simulink model "PF70mmDuctFanN"  (R2018b)
settings: Solver=FixedStepAuto  StartTime=0.0  StopTime=10.0  RelTol=1e-3
libraries: simulink x1, vrlib x1
settings Model: Creator=sweat  LastModifiedBy=39926

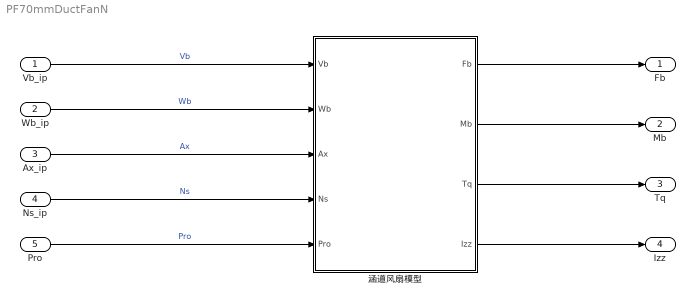
== system PF70mmDuctFanN ==
  Vb_ip : Inport  PortDimensions=3
  Wb_ip : Inport  Port=2  PortDimensions=3
  Ax_ip : Inport  Port=3  PortDimensions=3
  Ns_ip : Inport  Port=4  PortDimensions=1
  Pro : Inport  Port=5  PortDimensions=1
  "涵道风扇模型 " : Subsystem  mask{Fratio=1.016, Mratio=1.24, Izz=0.00000309}
      mask prompts: Fratio "涵道风扇气动力修正系数"; Mratio "涵道风扇气动力矩修正系数"; Izz "涵道风扇转动惯量"
  Fb : Outport
  Mb : Outport  Port=2
  Tq : Outport  Port=3
  Izz : Outport  Port=4
  wires:
  Vb_ip/1 -> "涵道风扇模型 "/1(Vb)  "Vb"
  Wb_ip/1 -> "涵道风扇模型 "/2(Wb)  "Wb"
  Ax_ip/1 -> "涵道风扇模型 "/3(Ax)  "Ax"
  Ns_ip/1 -> "涵道风扇模型 "/4(Ns)  "Ns"
  Pro/1 -> "涵道风扇模型 "/5(Pro)  "Pro"
  "涵道风扇模型 "/1(Fb) -> Fb/1
  "涵道风扇模型 "/2(Mb) -> Mb/1
  "涵道风扇模型 "/3(Tq) -> Tq/1
  "涵道风扇模型 "/4(Izz) -> Izz/1

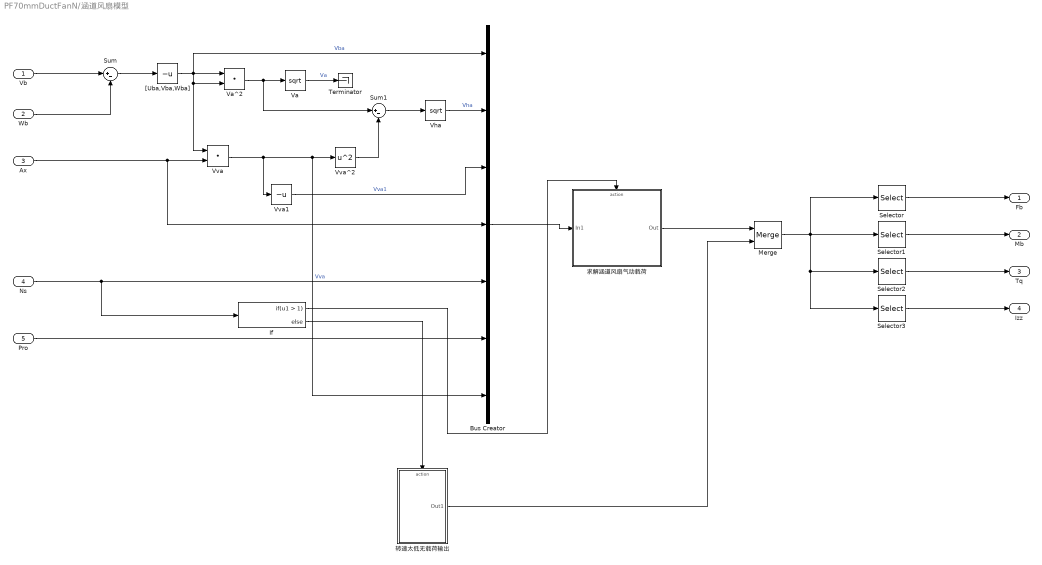
== system PF70mmDuctFanN/涵道风扇模型  ==
  Vb : Inport
  Wb : Inport  Port=2
  Ax : Inport  Port=3
  Ns : Inport  Port=4
  Pro : Inport  Port=5
  Bus Creator : BusCreator  Inputs=7
  If : If  IfExpression=u1 > 1
  Merge : Merge
  Selector : Selector  InputPortWidth=8  IndexOptions=Index vector (dialog)  Indices=[1:3]  OutputSizes=1
  Selector1 : Selector  InputPortWidth=8  IndexOptions=Index vector (dialog)  Indices=[4:6]  OutputSizes=1
  Selector2 : Selector  InputPortWidth=8  IndexOptions=Index vector (dialog)  Indices=[7]  OutputSizes=1
  Selector3 : Selector  InputPortWidth=8  IndexOptions=Index vector (dialog)  Indices=8  OutputSizes=1
  Sum : Sum  Inputs=|+-
  Sum1 : Sum  Inputs=|+-
  Terminator : Terminator
  Va : Sqrt  SaturateOnIntegerOverflow=on
  Va^2 : DotProduct  InputSameDT=on  OutDataTypeStr=Inherit: Inherit via internal rule
  Vha : Sqrt  SaturateOnIntegerOverflow=on
  Vva : DotProduct  InputSameDT=on  OutDataTypeStr=Inherit: Inherit via internal rule
  Vva1 : UnaryMinus
  Vva^2 : Math  Operator=square  SaturateOnIntegerOverflow=on
  "[Uba,Vba,Wba]" : UnaryMinus
  求解涵道风扇气动载荷 : Subsystem  TreatAsAtomicUnit=on
  转速太低无载荷输出 : Subsystem  TreatAsAtomicUnit=on
  Fb : Outport
  Mb : Outport  Port=2
  Tq : Outport  Port=3
  Izz : Outport  Port=4
  wires:
  Vb/1 -> Sum/1
  Wb/1 -> Sum/2
  Sum/1 -> "[Uba,Vba,Wba]"/1
  "[Uba,Vba,Wba]"/1 -> Bus Creator/1, Vva/1, Va^2/2, Va^2/1  "Vba"
  Ax/1 -> Bus Creator/4, Vva/2
  Va^2/1 -> Sum1/1, Va/1
  Vva/1 -> Bus Creator/7, Vva^2/1, Vva1/1  "Vva"
  Vva^2/1 -> Sum1/2
  Sum1/1 -> Vha/1
  Vha/1 -> Bus Creator/2  "Vha"
  Vva1/1 -> Bus Creator/3  "Vva1"
  Ns/1 -> Bus Creator/5, If/1
  If/1 -> 求解涵道风扇气动载荷/Action
  If/2 -> 转速太低无载荷输出/Action
  Pro/1 -> Bus Creator/6
  Bus Creator/1 -> 求解涵道风扇气动载荷/1(In1)
  Va/1 -> Terminator/1  "Va"
  Merge/1 -> Selector3/1, Selector2/1, Selector1/1, Selector/1
  求解涵道风扇气动载荷/1(Out) -> Merge/1
  转速太低无载荷输出/1(Out1) -> Merge/2
  Selector/1 -> Fb/1
  Selector1/1 -> Mb/1
  Selector2/1 -> Tq/1
  Selector3/1 -> Izz/1

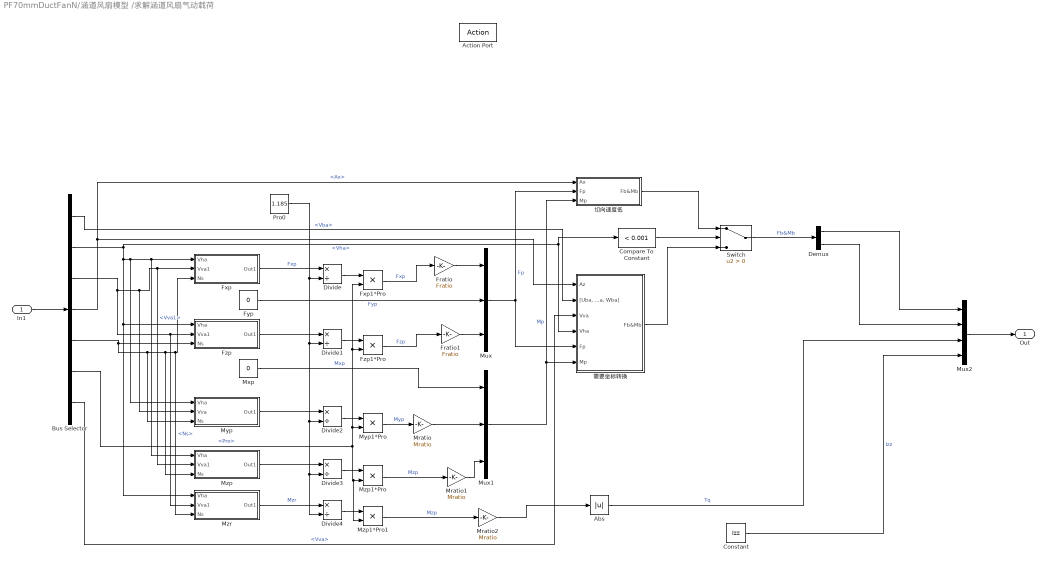
== system PF70mmDuctFanN/涵道风扇模型 /求解涵道风扇气动载荷 ==
  In1 : Inport
  Action Port : ActionPort  ActionType=then
  Abs : Abs
  Bus Selector : BusSelector  OutputSignals=Vba,Vha,Vva1,Ax,Ns,Pro,Vva
  Compare To Constant : simulink/Logic and Bit Operations/Compare To Constant  relop=<  const=0.001  OutDataTypeStr=boolean
  Constant : Constant  Value=Izz
  Demux : Demux  Outputs=2
  Divide{,1..4} (5 alike) : Product  Inputs=*/
  Fratio : Gain  Gain=Fratio
  Fratio1 : Gain  Gain=Fratio
  Fxp : Subsystem
  Fxp1*Pro : Product
  Fyp : Constant  Value=0
  Fzp : Subsystem
  Fzp1*Pro : Product
  Mratio : Gain  Gain=Mratio
  Mratio1 : Gain  Gain=Mratio
  Mratio2 : Gain  Gain=Mratio
  Mux : Mux  Inputs=3
  Mux1 : Mux  Inputs=3
  Mux2 : Mux
  Mxp : Constant  Value=0
  Myp : Subsystem
  Myp1*Pro : Product
  Mzp : Subsystem
  Mzp1*Pro : Product
  Mzp1*Pro1 : Product
  Mzr : Subsystem
  Pro0 : Constant  Value=1.185
  Switch : Switch  Criteria=u2 > Threshold
  切向速度低 : Subsystem
  需要坐标转换 : Subsystem
  Out : Outport
  wires:
  In1/1 -> Bus Selector/1
  Bus Selector/2 -> Mzr/1(Vha), Fzp/1(Vha), Myp/1(Vha), Mzp/1(Vha), Fxp/1(Vha), 需要坐标转换/4(Vha), Compare To Constant/1  "<Vha>"
  Bus Selector/3 -> Myp/2(Vva), Mzp/2(Vva1), Fxp/2(Vva1), Mzr/2(Vva1), Fzp/2(Vva1)  "<Vva1>"
  Bus Selector/5 -> Fzp/3(Ns), Myp/3(Ns), Mzp/3(Ns), Mzr/3(Ns), Fxp/3(Ns)  "<Ns>"
  Fyp/1 -> Mux/2  "Fyp"
  Fxp/1(Out1) -> Divide/1  "Fxp"
  Fzp/1(Out1) -> Divide1/1
  Myp/1(Out1) -> Divide2/1
  Mzp/1(Out1) -> Divide3/1
  Pro0/1 -> Divide4/2, Divide3/2, Divide2/2, Divide1/2, Divide/2
  Divide/1 -> Fxp1*Pro/1
  Fxp1*Pro/1 -> Fratio/1  "Fxp"
  Divide1/1 -> Fzp1*Pro/1
  Fzp1*Pro/1 -> Fratio1/1  "Fzp"
  Bus Selector/6 -> Mzp1*Pro1/2, Mzp1*Pro/2, Myp1*Pro/2, Fzp1*Pro/2, Fxp1*Pro/2  "<Pro>"
  Divide2/1 -> Myp1*Pro/1
  Myp1*Pro/1 -> Mratio/1  "Myp"
  Divide3/1 -> Mzp1*Pro/1
  Bus Selector/4 -> 需要坐标转换/1(Az), 切向速度低/1(Ax)  "<Ax>"
  Mux/1 -> 需要坐标转换/5(Fp), 切向速度低/2(Fp)  "Fp"
  Mux1/1 -> 需要坐标转换/6(Mp), 切向速度低/3(Mp)  "Mp"
  Bus Selector/1 -> 需要坐标转换/2("[Uba, Vba, Wba]")  "<Vba>"
  Bus Selector/7 -> 需要坐标转换/3(Vva)  "<Vva>"
  Compare To Constant/1 -> Switch/2
  需要坐标转换/1(Fb&Mb) -> Switch/3
  Abs/1 -> Mux2/3  "Tq"
  Mzp1*Pro/1 -> Mratio1/1  "Mzp"
  Fratio/1 -> Mux/1
  Fratio1/1 -> Mux/3
  Mratio/1 -> Mux1/2
  Mratio2/1 -> Abs/1
  Constant/1 -> Mux2/4  "Izz"
  Switch/1 -> Demux/1  "Fb&Mb"
  切向速度低/1(Fb&Mb) -> Switch/1
  Mxp/1 -> Mux1/1  "Mxp"
  Mzr/1(Out1) -> Divide4/1  "Mzr"
  Divide4/1 -> Mzp1*Pro1/1
  Mzp1*Pro1/1 -> Mratio2/1  "Mzp"
  Mratio1/1 -> Mux1/3
  Mux2/1 -> Out/1
  Demux/2 -> Mux2/2
  Demux/1 -> Mux2/1

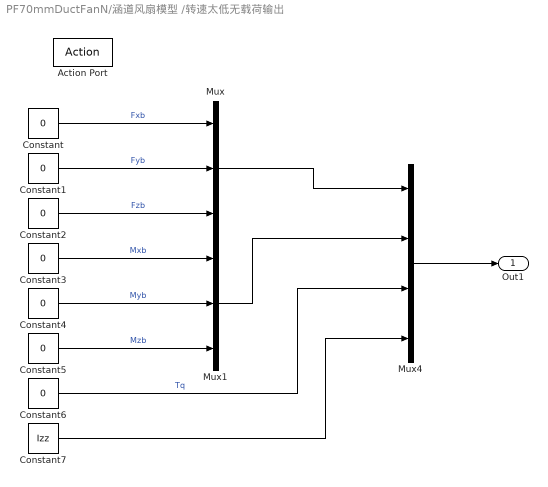
== system PF70mmDuctFanN/涵道风扇模型 /转速太低无载荷输出 ==
  Action Port : ActionPort  ActionType=else
  Constant{,1..6} (7 alike) : Constant  Value=0
  Constant7 : Constant  Value=Izz
  Mux : Mux  Inputs=3
  Mux1 : Mux  Inputs=3
  Mux4 : Mux
  Out1 : Outport
  wires:
  Constant/1 -> Mux/1  "Fxb"
  Constant1/1 -> Mux/2  "Fyb"
  Constant2/1 -> Mux/3  "Fzb"
  Constant3/1 -> Mux1/1  "Mxb"
  Constant4/1 -> Mux1/2  "Myb"
  Constant5/1 -> Mux1/3  "Mzb"
  Constant6/1 -> Mux4/3  "Tq"
  Mux/1 -> Mux4/1
  Constant7/1 -> Mux4/4
  Mux1/1 -> Mux4/2
  Mux4/1 -> Out1/1

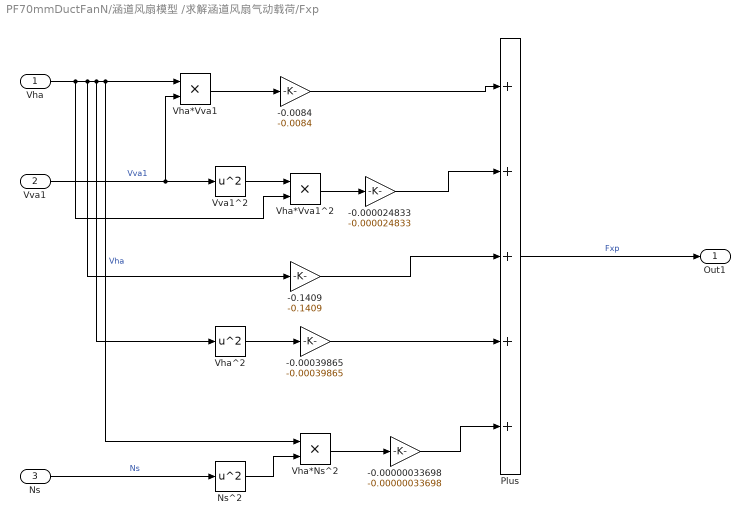
== system PF70mmDuctFanN/涵道风扇模型 /求解涵道风扇气动载荷/Fxp ==
  Vha : Inport
  Vva1 : Inport  Port=2
  Ns : Inport  Port=3
  -0.00000033698 : Gain  Gain=-0.00000033698
  -0.000024833 : Gain  Gain=-0.000024833
  -0.00039865 : Gain  Gain=-0.00039865
  -0.0084 : Gain  Gain=-0.0084
  -0.1409 : Gain  Gain=-0.1409
  Ns^2 : Math  Operator=square  SaturateOnIntegerOverflow=on
  Plus : Sum  Inputs=+++++
  Vha*Ns^2 : Product
  Vha*Vva1 : Product
  Vha*Vva1^2 : Product
  Vha^2 : Math  Operator=square  SaturateOnIntegerOverflow=on
  Vva1^2 : Math  Operator=square  SaturateOnIntegerOverflow=on
  Out1 : Outport
  wires:
  Vha/1 -> Vha*Vva1^2/2, -0.1409/1, Vha^2/1, Vha*Ns^2/1, Vha*Vva1/1  "Vha"
  Vva1/1 -> Vva1^2/1, Vha*Vva1/2  "Vva1"
  Vha*Vva1/1 -> -0.0084/1
  -0.0084/1 -> Plus/1
  Ns/1 -> Ns^2/1  "Ns"
  Vva1^2/1 -> Vha*Vva1^2/1
  Vha*Vva1^2/1 -> -0.000024833/1
  -0.000024833/1 -> Plus/2
  -0.1409/1 -> Plus/3
  Vha^2/1 -> -0.00039865/1
  -0.00039865/1 -> Plus/4
  Ns^2/1 -> Vha*Ns^2/2
  Vha*Ns^2/1 -> -0.00000033698/1
  -0.00000033698/1 -> Plus/5
  Plus/1 -> Out1/1  "Fxp"

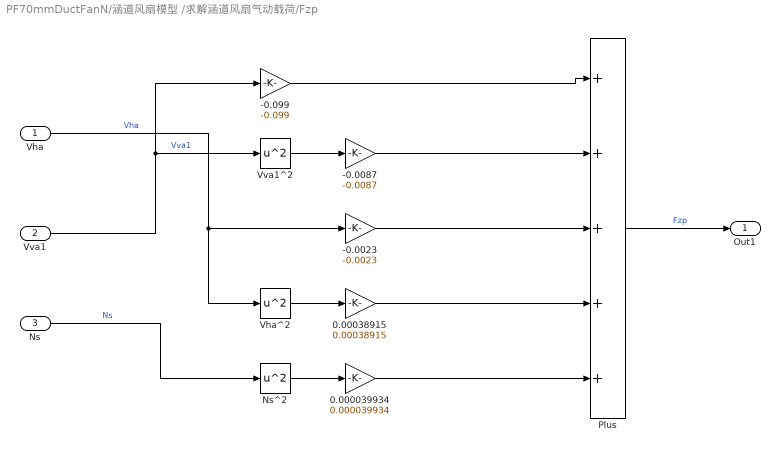
== system PF70mmDuctFanN/涵道风扇模型 /求解涵道风扇气动载荷/Fzp ==
  Vha : Inport
  Vva1 : Inport  Port=2
  Ns : Inport  Port=3
  -0.0023 : Gain  Gain=-0.0023
  -0.0087 : Gain  Gain=-0.0087
  -0.099 : Gain  Gain=-0.099
  0.000039934 : Gain  Gain=0.000039934
  0.00038915 : Gain  Gain=0.00038915
  Ns^2 : Math  Operator=square  SaturateOnIntegerOverflow=on
  Plus : Sum  Inputs=+++++
  Vha^2 : Math  Operator=square  SaturateOnIntegerOverflow=on
  Vva1^2 : Math  Operator=square  SaturateOnIntegerOverflow=on
  Out1 : Outport
  wires:
  Vha/1 -> Vha^2/1, -0.0023/1  "Vha"
  Vva1/1 -> -0.099/1, Vva1^2/1  "Vva1"
  Ns/1 -> Ns^2/1  "Ns"
  -0.099/1 -> Plus/1
  Vva1^2/1 -> -0.0087/1
  -0.0087/1 -> Plus/2
  Vha^2/1 -> 0.00038915/1
  Ns^2/1 -> 0.000039934/1
  0.000039934/1 -> Plus/5
  Plus/1 -> Out1/1  "Fzp"
  -0.0023/1 -> Plus/3
  0.00038915/1 -> Plus/4

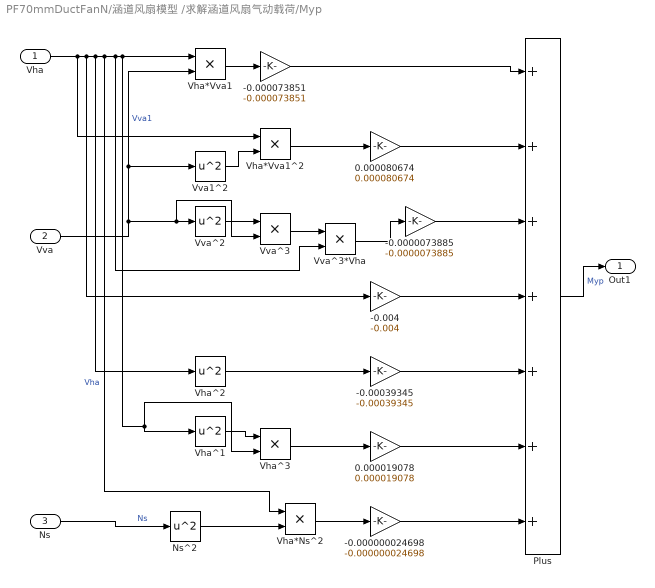
== system PF70mmDuctFanN/涵道风扇模型 /求解涵道风扇气动载荷/Myp ==
  Vha : Inport
  Vva : Inport  Port=2
  Ns : Inport  Port=3
  -0.000000024698 : Gain  Gain=-0.000000024698
  -0.0000073885 : Gain  Gain=-0.0000073885
  -0.000073851 : Gain  Gain=-0.000073851
  -0.00039345 : Gain  Gain=-0.00039345
  -0.004 : Gain  Gain=-0.004
  0.000019078 : Gain  Gain=0.000019078
  0.000080674 : Gain  Gain=0.000080674
  Ns^2 : Math  Operator=square  SaturateOnIntegerOverflow=on
  Plus : Sum  Inputs=+++++++
  Vha*Ns^2 : Product
  Vha*Vva1 : Product
  Vha*Vva1^2 : Product
  Vha^1 : Math  Operator=square  SaturateOnIntegerOverflow=on
  Vha^2 : Math  Operator=square  SaturateOnIntegerOverflow=on
  Vha^3 : Product
  Vva1^2 : Math  Operator=square  SaturateOnIntegerOverflow=on
  Vva^2 : Math  Operator=square  SaturateOnIntegerOverflow=on
  Vva^3 : Product
  Vva^3*Vha : Product
  Out1 : Outport
  wires:
  Vha/1 -> Vha*Vva1^2/1, -0.004/1, Vha^2/1, Vha*Ns^2/1, Vha^3/2, Vha^1/1, Vha*Vva1/1, Vva^3*Vha/2  "Vha"
  Vva/1 -> Vha*Vva1/2, Vva1^2/1, Vva^3/2, Vva^2/1  "Vva1"
  Ns/1 -> Ns^2/1  "Ns"
  Plus/1 -> Out1/1  "Myp"
  Vha*Vva1/1 -> -0.000073851/1
  -0.000073851/1 -> Plus/1
  Vha*Vva1^2/1 -> 0.000080674/1
  0.000080674/1 -> Plus/2
  Vva1^2/1 -> Vha*Vva1^2/2
  -0.004/1 -> Plus/4
  Vha^2/1 -> -0.00039345/1
  -0.00039345/1 -> Plus/5
  Vha*Ns^2/1 -> -0.000000024698/1
  Ns^2/1 -> Vha*Ns^2/2
  Vha^1/1 -> Vha^3/1
  Vha^3/1 -> 0.000019078/1
  -0.000000024698/1 -> Plus/7
  0.000019078/1 -> Plus/6
  Vva^2/1 -> Vva^3/1
  Vva^3/1 -> Vva^3*Vha/1
  Vva^3*Vha/1 -> -0.0000073885/1
  -0.0000073885/1 -> Plus/3

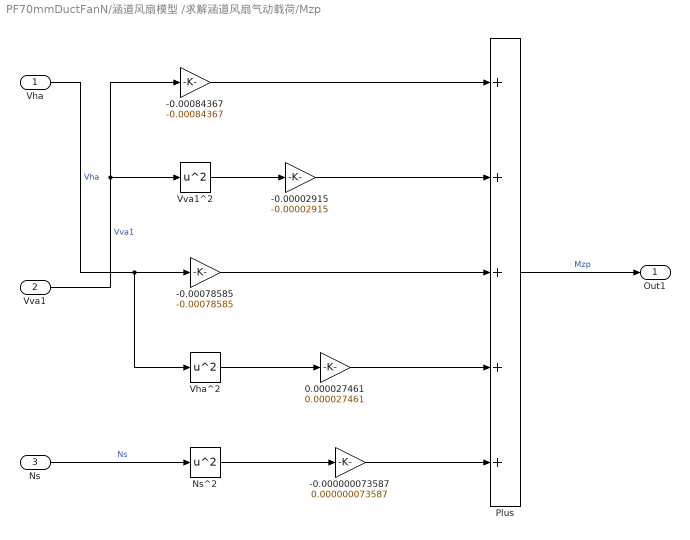
== system PF70mmDuctFanN/涵道风扇模型 /求解涵道风扇气动载荷/Mzp ==
  Vha : Inport
  Vva1 : Inport  Port=2
  Ns : Inport  Port=3
  "-0.000000073587 " : Gain  Gain=0.000000073587
  -0.00002915 : Gain  Gain=-0.00002915
  -0.00078585 : Gain  Gain=-0.00078585
  -0.00084367 : Gain  Gain=-0.00084367
  0.000027461 : Gain  Gain=0.000027461
  Ns^2 : Math  Operator=square  SaturateOnIntegerOverflow=on
  Plus : Sum  Inputs=+++++
  Vha^2 : Math  Operator=square  SaturateOnIntegerOverflow=on
  Vva1^2 : Math  Operator=square  SaturateOnIntegerOverflow=on
  Out1 : Outport
  wires:
  Plus/1 -> Out1/1  "Mzp"
  Vha/1 -> Vha^2/1, -0.00078585/1  "Vha"
  Vva1/1 -> Vva1^2/1, -0.00084367/1  "Vva1"
  Ns/1 -> Ns^2/1  "Ns"
  -0.00084367/1 -> Plus/1
  -0.00002915/1 -> Plus/2
  Vva1^2/1 -> -0.00002915/1
  -0.00078585/1 -> Plus/3
  0.000027461/1 -> Plus/4
  Vha^2/1 -> 0.000027461/1
  "-0.000000073587 "/1 -> Plus/5
  Ns^2/1 -> "-0.000000073587 "/1

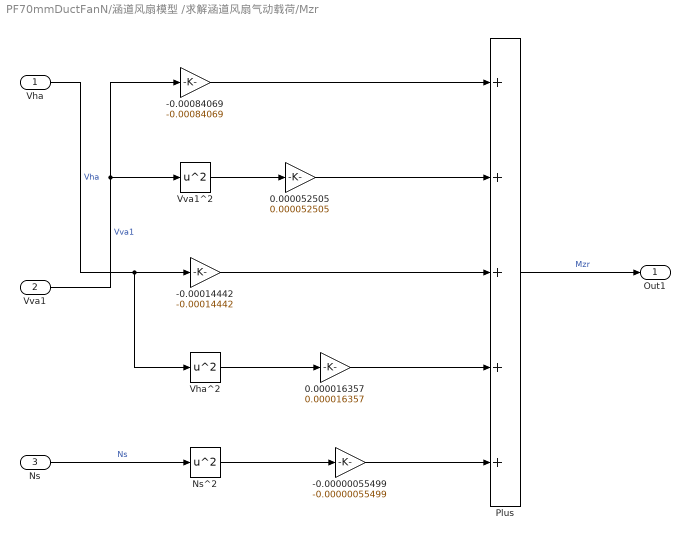
== system PF70mmDuctFanN/涵道风扇模型 /求解涵道风扇气动载荷/Mzr ==
  Vha : Inport
  Vva1 : Inport  Port=2
  Ns : Inport  Port=3
  "-0.00000055499 " : Gain  Gain=-0.00000055499
  -0.00014442 : Gain  Gain=-0.00014442
  -0.00084069 : Gain  Gain=-0.00084069
  0.000016357 : Gain  Gain=0.000016357
  0.000052505 : Gain  Gain=0.000052505
  Ns^2 : Math  Operator=square  SaturateOnIntegerOverflow=on
  Plus : Sum  Inputs=+++++
  Vha^2 : Math  Operator=square  SaturateOnIntegerOverflow=on
  Vva1^2 : Math  Operator=square  SaturateOnIntegerOverflow=on
  Out1 : Outport
  wires:
  Plus/1 -> Out1/1  "Mzr"
  Vha/1 -> Vha^2/1, -0.00014442/1  "Vha"
  Vva1/1 -> Vva1^2/1, -0.00084069/1  "Vva1"
  Ns/1 -> Ns^2/1  "Ns"
  -0.00084069/1 -> Plus/1
  0.000052505/1 -> Plus/2
  Vva1^2/1 -> 0.000052505/1
  -0.00014442/1 -> Plus/3
  0.000016357/1 -> Plus/4
  Vha^2/1 -> 0.000016357/1
  "-0.00000055499 "/1 -> Plus/5
  Ns^2/1 -> "-0.00000055499 "/1

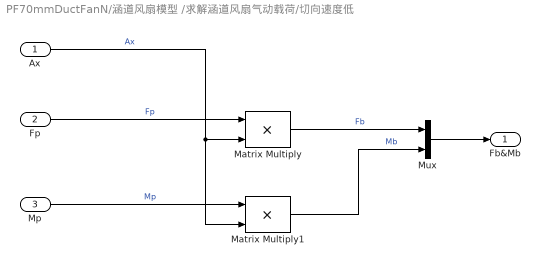
== system PF70mmDuctFanN/涵道风扇模型 /求解涵道风扇气动载荷/切向速度低 ==
  Ax : Inport
  Fp : Inport  Port=2
  Mp : Inport  Port=3
  Matrix Multiply : Product
  Matrix Multiply1 : Product
  Mux : Mux  Inputs=2
  Fb&Mb : Outport
  wires:
  Ax/1 -> Matrix Multiply1/2, Matrix Multiply/2  "Ax"
  Fp/1 -> Matrix Multiply/1  "Fp"
  Mp/1 -> Matrix Multiply1/1  "Mp"
  Mux/1 -> Fb&Mb/1
  Matrix Multiply/1 -> Mux/1  "Fb"
  Matrix Multiply1/1 -> Mux/2  "Mb"

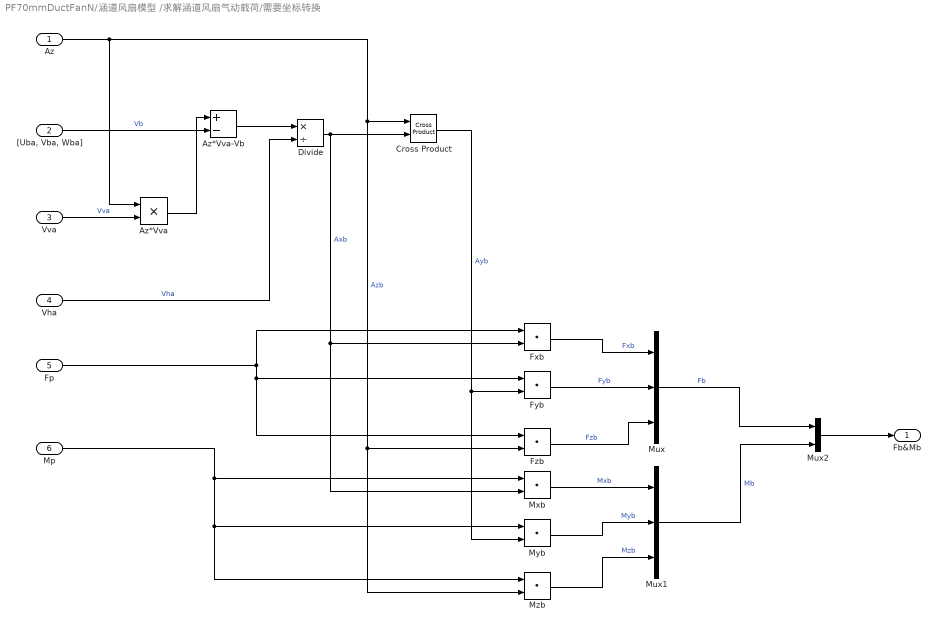
== system PF70mmDuctFanN/涵道风扇模型 /求解涵道风扇气动载荷/需要坐标转换 ==
  Az : Inport
  "[Uba, Vba, Wba]" : Inport  Port=2
  Vva : Inport  Port=3
  Vha : Inport  Port=4
  Fp : Inport  Port=5
  Mp : Inport  Port=6
  Az*Vva : Product
  Az*Vva-Vb : Sum  Inputs=+-
  Cross Product : vrlib/Utilities/Cross Product
      settings: SourceProductBaseCode=VR
  Divide : Product  Inputs=*/
  Fxb : DotProduct  InputSameDT=on  OutDataTypeStr=Inherit: Inherit via internal rule
  Fyb : DotProduct  InputSameDT=on  OutDataTypeStr=Inherit: Inherit via internal rule
  Fzb : DotProduct  InputSameDT=on  OutDataTypeStr=Inherit: Inherit via internal rule
  Mux : Mux  Inputs=3
  Mux1 : Mux  Inputs=3
  Mux2 : Mux  Inputs=2
  Mxb : DotProduct  InputSameDT=on  OutDataTypeStr=Inherit: Inherit via internal rule
  Myb : DotProduct  InputSameDT=on  OutDataTypeStr=Inherit: Inherit via internal rule
  Mzb : DotProduct  InputSameDT=on  OutDataTypeStr=Inherit: Inherit via internal rule
  Fb&Mb : Outport
  wires:
  Vva/1 -> Az*Vva/2  "Vva"
  Az/1 -> Cross Product/1, Fzb/2, Mzb/2, Az*Vva/1  "Azb"
  Az*Vva/1 -> Az*Vva-Vb/1
  "[Uba, Vba, Wba]"/1 -> Az*Vva-Vb/2  "Vb"
  Az*Vva-Vb/1 -> Divide/1
  Vha/1 -> Divide/2  "Vha"
  Divide/1 -> Cross Product/2, Mxb/2, Fxb/2  "Axb"
  Cross Product/1 -> Myb/2, Fyb/2  "Ayb"
  Fp/1 -> Fzb/1, Fyb/1, Fxb/1
  Mp/1 -> Mzb/1, Myb/1, Mxb/1
  Fxb/1 -> Mux/1  "Fxb"
  Fyb/1 -> Mux/2  "Fyb"
  Fzb/1 -> Mux/3  "Fzb"
  Mxb/1 -> Mux1/1  "Mxb"
  Myb/1 -> Mux1/2  "Myb"
  Mzb/1 -> Mux1/3  "Mzb"
  Mux/1 -> Mux2/1  "Fb"
  Mux1/1 -> Mux2/2  "Mb"
  Mux2/1 -> Fb&Mb/1
